simulink model "EEL_5661_F22_tricycle_100322"  (R2019a)
settings: Solver=VariableStepAuto  StartTime=0.0  StopTime=10.0  RelTol=1e-3
libraries: simulink x1
settings Model: Creator=rothz  LastModifiedBy=rothz

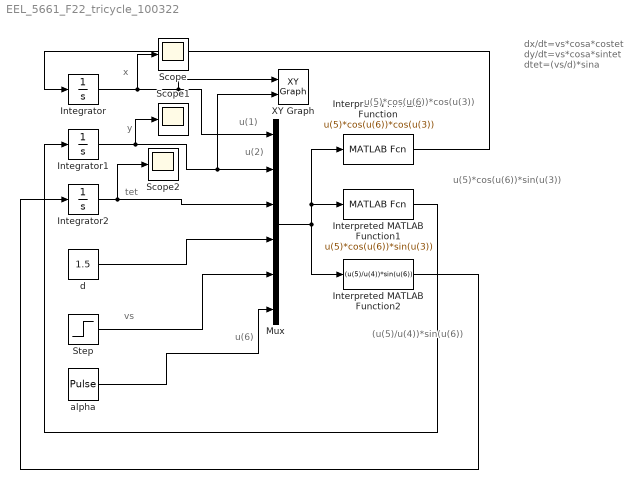
== system EEL_5661_F22_tricycle_100322 ==
  note: (u(5)/u(4))*sin(u(6))
  note: u(5)*cos(u(6))*sin(u(3))
  note: u(5)*cos(u(6))*cos(u(3))
  note: u(6)
  note: u(2)
  note: u(1)
  note: vs
  note: tet
  note: y
  note: x
  note: dx/dt=vs*cosa*costet
      | dy/dt=vs*cosa*sintet
      | dtet=(vs/d)*sina
  Integrator : Integrator
  Integrator1 : Integrator
  Integrator2 : Integrator
  Interpreted MATLAB Function : MATLABFcn  MATLABFcn=u(5)*cos(u(6))*cos(u(3))  OutputDimensions=1
  Interpreted MATLAB Function1 : MATLABFcn  MATLABFcn=u(5)*cos(u(6))*sin(u(3))  OutputDimensions=1
  Interpreted MATLAB Function2 : MATLABFcn  MATLABFcn=(u(5)/u(4))*sin(u(6))  OutputDimensions=1
  Mux : Mux  Inputs=6
  Scope : Scope
  Scope1 : Scope
  Scope2 : Scope
  Step : Step  SampleTime=0
  XY Graph : simulink/Sinks/XY Graph  xmin=-1  xmax=10  ymin=-1  ymax=5  st=-1
  alpha : DiscretePulseGenerator  PulseType=Time based  Amplitude=0.5  Period=20  PulseWidth=5  PhaseDelay=2
  d : Constant  Value=1.5
  wires:
  Integrator/1 -> Scope/1, XY Graph/1, Mux/1
  Integrator1/1 -> Scope1/1, XY Graph/2, Mux/2
  Integrator2/1 -> Scope2/1, Mux/3
  d/1 -> Mux/4
  Step/1 -> Mux/5
  alpha/1 -> Mux/6
  Mux/1 -> Interpreted MATLAB Function1/1, Interpreted MATLAB Function/1, Interpreted MATLAB Function2/1
  Interpreted MATLAB Function/1 -> Integrator/1
  Interpreted MATLAB Function1/1 -> Integrator1/1
  Interpreted MATLAB Function2/1 -> Integrator2/1
